simulink model "gm_test_cost_function_only_without_delays"  (R2022a)
settings: Solver=FixedStepDiscrete  StartTime=0.0  StopTime=10.0  RelTol=1e-3
undefined symbols (not defined in the file or in its folder): f_c
libraries: hdlmdlgenlib x64
(part 2 of 2)

== system gm_test_cost_function_only_without_delays/HDL_DUT1/Subsystem/Subsystem4 ==
  Prediction_5 : Inport  OutDataTypeStr=fixdt(1, 18, 11)  PortDimensions=[4]  SampleTime=1e-08
  id_ref : Inport  Port=2  OutDataTypeStr=fixdt(1, 18, 11)  PortDimensions=1  SampleTime=1e-08
  iq_ref : Inport  Port=3  OutDataTypeStr=fixdt(1, 18, 11)  PortDimensions=1  SampleTime=1e-08
  ix_ref : Inport  Port=4  OutDataTypeStr=fixdt(1, 18, 11)  PortDimensions=1  SampleTime=1e-08
  iy_ref : Inport  Port=5  OutDataTypeStr=fixdt(1, 18, 11)  PortDimensions=1  SampleTime=1e-08
  Prediction_5_0_wire : hdlmdlgenlib/Buffer
      settings: SourceProductBaseCode=SL
  Prediction_5_1_wire : hdlmdlgenlib/Buffer
      settings: SourceProductBaseCode=SL
  Prediction_5_2_wire : hdlmdlgenlib/Buffer
      settings: SourceProductBaseCode=SL
  Prediction_5_3_wire : hdlmdlgenlib/Buffer
      settings: SourceProductBaseCode=SL
  Product{1..4} (4 alike) : Product  Inputs=**  OutDataTypeStr=fixdt(1, 20, 11)  SampleTime=1e-08
  Subtract{4..7} (4 alike) : Sum  Inputs=+-  AccumDataTypeStr=fixdt(1, 19, 11)  OutDataTypeStr=fixdt(1, 20, 11)  SampleTime=1e-08
  Sum of Elements_stage2 : Sum  AccumDataTypeStr=fixdt(1, 22, 11)  OutDataTypeStr=fixdt(1, 21, 11)  SampleTime=1e-08
  Sum of Elements_stage3 : Sum  AccumDataTypeStr=fixdt(1, 22, 11)  OutDataTypeStr=fixdt(1, 22, 11)  SampleTime=1e-08
  Sum of Elements_stage4 : Sum  AccumDataTypeStr=fixdt(1, 22, 11)  OutDataTypeStr=fixdt(1, 20, 11)  SampleTime=1e-08
  t : Demux
  J5 : Outport  SampleTime=1e-08
  wires:
  Prediction_5/1 -> t/1
  id_ref/1 -> Subtract4/1
  iq_ref/1 -> Subtract5/1
  ix_ref/1 -> Subtract6/1
  iy_ref/1 -> Subtract7/1
  Prediction_5_0_wire/1 -> Subtract4/2
  Prediction_5_1_wire/1 -> Subtract5/2
  Prediction_5_2_wire/1 -> Subtract6/2
  Prediction_5_3_wire/1 -> Subtract7/2
  Product1/1 -> Sum of Elements_stage2/2
  Product2/1 -> Sum of Elements_stage3/2
  Product3/1 -> Sum of Elements_stage2/1
  Product4/1 -> Sum of Elements_stage4/2
  Subtract4/1 -> Product3/2, Product3/1
  Subtract5/1 -> Product1/2, Product1/1
  Subtract6/1 -> Product2/2, Product2/1
  Subtract7/1 -> Product4/2, Product4/1
  Sum of Elements_stage4/1 -> J5/1
  t/1 -> Prediction_5_0_wire/1
  t/2 -> Prediction_5_1_wire/1
  t/3 -> Prediction_5_2_wire/1
  t/4 -> Prediction_5_3_wire/1
  Sum of Elements_stage2/1 -> Sum of Elements_stage3/1
  Sum of Elements_stage3/1 -> Sum of Elements_stage4/1

== system gm_test_cost_function_only_without_delays/HDL_DUT1/Subsystem/Subsystem5 ==
  Prediction_6 : Inport  OutDataTypeStr=fixdt(1, 18, 11)  PortDimensions=[4]  SampleTime=1e-08
  id_ref : Inport  Port=2  OutDataTypeStr=fixdt(1, 18, 11)  PortDimensions=1  SampleTime=1e-08
  iq_ref : Inport  Port=3  OutDataTypeStr=fixdt(1, 18, 11)  PortDimensions=1  SampleTime=1e-08
  ix_ref : Inport  Port=4  OutDataTypeStr=fixdt(1, 18, 11)  PortDimensions=1  SampleTime=1e-08
  iy_ref : Inport  Port=5  OutDataTypeStr=fixdt(1, 18, 11)  PortDimensions=1  SampleTime=1e-08
  Prediction_6_0_wire : hdlmdlgenlib/Buffer
      settings: SourceProductBaseCode=SL
  Prediction_6_1_wire : hdlmdlgenlib/Buffer
      settings: SourceProductBaseCode=SL
  Prediction_6_2_wire : hdlmdlgenlib/Buffer
      settings: SourceProductBaseCode=SL
  Prediction_6_3_wire : hdlmdlgenlib/Buffer
      settings: SourceProductBaseCode=SL
  Product{1..4} (4 alike) : Product  Inputs=**  OutDataTypeStr=fixdt(1, 20, 11)  SampleTime=1e-08
  Subtract{4..7} (4 alike) : Sum  Inputs=+-  AccumDataTypeStr=fixdt(1, 19, 11)  OutDataTypeStr=fixdt(1, 20, 11)  SampleTime=1e-08
  Sum of Elements_stage2 : Sum  AccumDataTypeStr=fixdt(1, 22, 11)  OutDataTypeStr=fixdt(1, 21, 11)  SampleTime=1e-08
  Sum of Elements_stage3 : Sum  AccumDataTypeStr=fixdt(1, 22, 11)  OutDataTypeStr=fixdt(1, 22, 11)  SampleTime=1e-08
  Sum of Elements_stage4 : Sum  AccumDataTypeStr=fixdt(1, 22, 11)  OutDataTypeStr=fixdt(1, 20, 11)  SampleTime=1e-08
  t : Demux
  J6 : Outport  SampleTime=1e-08
  wires:
  Prediction_6/1 -> t/1
  id_ref/1 -> Subtract4/1
  iq_ref/1 -> Subtract5/1
  ix_ref/1 -> Subtract6/1
  iy_ref/1 -> Subtract7/1
  Prediction_6_0_wire/1 -> Subtract4/2
  Prediction_6_1_wire/1 -> Subtract5/2
  Prediction_6_2_wire/1 -> Subtract6/2
  Prediction_6_3_wire/1 -> Subtract7/2
  Product1/1 -> Sum of Elements_stage2/2
  Product2/1 -> Sum of Elements_stage3/2
  Product3/1 -> Sum of Elements_stage2/1
  Product4/1 -> Sum of Elements_stage4/2
  Subtract4/1 -> Product3/2, Product3/1
  Subtract5/1 -> Product1/2, Product1/1
  Subtract6/1 -> Product2/2, Product2/1
  Subtract7/1 -> Product4/2, Product4/1
  Sum of Elements_stage4/1 -> J6/1
  t/1 -> Prediction_6_0_wire/1
  t/2 -> Prediction_6_1_wire/1
  t/3 -> Prediction_6_2_wire/1
  t/4 -> Prediction_6_3_wire/1
  Sum of Elements_stage2/1 -> Sum of Elements_stage3/1
  Sum of Elements_stage3/1 -> Sum of Elements_stage4/1

== system gm_test_cost_function_only_without_delays/HDL_DUT1/Subsystem/Subsystem6 ==
  Prediction_7 : Inport  OutDataTypeStr=fixdt(1, 18, 11)  PortDimensions=[4]  SampleTime=1e-08
  id_ref : Inport  Port=2  OutDataTypeStr=fixdt(1, 18, 11)  PortDimensions=1  SampleTime=1e-08
  iq_ref : Inport  Port=3  OutDataTypeStr=fixdt(1, 18, 11)  PortDimensions=1  SampleTime=1e-08
  ix_ref : Inport  Port=4  OutDataTypeStr=fixdt(1, 18, 11)  PortDimensions=1  SampleTime=1e-08
  iy_ref : Inport  Port=5  OutDataTypeStr=fixdt(1, 18, 11)  PortDimensions=1  SampleTime=1e-08
  Prediction_7_0_wire : hdlmdlgenlib/Buffer
      settings: SourceProductBaseCode=SL
  Prediction_7_1_wire : hdlmdlgenlib/Buffer
      settings: SourceProductBaseCode=SL
  Prediction_7_2_wire : hdlmdlgenlib/Buffer
      settings: SourceProductBaseCode=SL
  Prediction_7_3_wire : hdlmdlgenlib/Buffer
      settings: SourceProductBaseCode=SL
  Product{1..4} (4 alike) : Product  Inputs=**  OutDataTypeStr=fixdt(1, 20, 11)  SampleTime=1e-08
  Subtract{4..7} (4 alike) : Sum  Inputs=+-  AccumDataTypeStr=fixdt(1, 19, 11)  OutDataTypeStr=fixdt(1, 20, 11)  SampleTime=1e-08
  Sum of Elements_stage2 : Sum  AccumDataTypeStr=fixdt(1, 22, 11)  OutDataTypeStr=fixdt(1, 21, 11)  SampleTime=1e-08
  Sum of Elements_stage3 : Sum  AccumDataTypeStr=fixdt(1, 22, 11)  OutDataTypeStr=fixdt(1, 22, 11)  SampleTime=1e-08
  Sum of Elements_stage4 : Sum  AccumDataTypeStr=fixdt(1, 22, 11)  OutDataTypeStr=fixdt(1, 20, 11)  SampleTime=1e-08
  t : Demux
  J7 : Outport  SampleTime=1e-08
  wires:
  Prediction_7/1 -> t/1
  id_ref/1 -> Subtract4/1
  iq_ref/1 -> Subtract5/1
  ix_ref/1 -> Subtract6/1
  iy_ref/1 -> Subtract7/1
  Prediction_7_0_wire/1 -> Subtract4/2
  Prediction_7_1_wire/1 -> Subtract5/2
  Prediction_7_2_wire/1 -> Subtract6/2
  Prediction_7_3_wire/1 -> Subtract7/2
  Product1/1 -> Sum of Elements_stage2/2
  Product2/1 -> Sum of Elements_stage3/2
  Product3/1 -> Sum of Elements_stage2/1
  Product4/1 -> Sum of Elements_stage4/2
  Subtract4/1 -> Product3/2, Product3/1
  Subtract5/1 -> Product1/2, Product1/1
  Subtract6/1 -> Product2/2, Product2/1
  Subtract7/1 -> Product4/2, Product4/1
  Sum of Elements_stage4/1 -> J7/1
  t/1 -> Prediction_7_0_wire/1
  t/2 -> Prediction_7_1_wire/1
  t/3 -> Prediction_7_2_wire/1
  t/4 -> Prediction_7_3_wire/1
  Sum of Elements_stage2/1 -> Sum of Elements_stage3/1
  Sum of Elements_stage3/1 -> Sum of Elements_stage4/1

== system gm_test_cost_function_only_without_delays/HDL_DUT1/Subsystem/Subsystem7 ==
  Prediction_8 : Inport  OutDataTypeStr=fixdt(1, 18, 11)  PortDimensions=[4]  SampleTime=1e-08
  id_ref : Inport  Port=2  OutDataTypeStr=fixdt(1, 18, 11)  PortDimensions=1  SampleTime=1e-08
  iq_ref : Inport  Port=3  OutDataTypeStr=fixdt(1, 18, 11)  PortDimensions=1  SampleTime=1e-08
  ix_ref : Inport  Port=4  OutDataTypeStr=fixdt(1, 18, 11)  PortDimensions=1  SampleTime=1e-08
  iy_ref : Inport  Port=5  OutDataTypeStr=fixdt(1, 18, 11)  PortDimensions=1  SampleTime=1e-08
  Prediction_8_0_wire : hdlmdlgenlib/Buffer
      settings: SourceProductBaseCode=SL
  Prediction_8_1_wire : hdlmdlgenlib/Buffer
      settings: SourceProductBaseCode=SL
  Prediction_8_2_wire : hdlmdlgenlib/Buffer
      settings: SourceProductBaseCode=SL
  Prediction_8_3_wire : hdlmdlgenlib/Buffer
      settings: SourceProductBaseCode=SL
  Product{1..4} (4 alike) : Product  Inputs=**  OutDataTypeStr=fixdt(1, 20, 11)  SampleTime=1e-08
  Subtract{4..7} (4 alike) : Sum  Inputs=+-  AccumDataTypeStr=fixdt(1, 19, 11)  OutDataTypeStr=fixdt(1, 20, 11)  SampleTime=1e-08
  Sum of Elements_stage2 : Sum  AccumDataTypeStr=fixdt(1, 22, 11)  OutDataTypeStr=fixdt(1, 21, 11)  SampleTime=1e-08
  Sum of Elements_stage3 : Sum  AccumDataTypeStr=fixdt(1, 22, 11)  OutDataTypeStr=fixdt(1, 22, 11)  SampleTime=1e-08
  Sum of Elements_stage4 : Sum  AccumDataTypeStr=fixdt(1, 22, 11)  OutDataTypeStr=fixdt(1, 20, 11)  SampleTime=1e-08
  t : Demux
  J8 : Outport  SampleTime=1e-08
  wires:
  Prediction_8/1 -> t/1
  id_ref/1 -> Subtract4/1
  iq_ref/1 -> Subtract5/1
  ix_ref/1 -> Subtract6/1
  iy_ref/1 -> Subtract7/1
  Prediction_8_0_wire/1 -> Subtract4/2
  Prediction_8_1_wire/1 -> Subtract5/2
  Prediction_8_2_wire/1 -> Subtract6/2
  Prediction_8_3_wire/1 -> Subtract7/2
  Product1/1 -> Sum of Elements_stage2/2
  Product2/1 -> Sum of Elements_stage3/2
  Product3/1 -> Sum of Elements_stage2/1
  Product4/1 -> Sum of Elements_stage4/2
  Subtract4/1 -> Product3/2, Product3/1
  Subtract5/1 -> Product1/2, Product1/1
  Subtract6/1 -> Product2/2, Product2/1
  Subtract7/1 -> Product4/2, Product4/1
  Sum of Elements_stage4/1 -> J8/1
  t/1 -> Prediction_8_0_wire/1
  t/2 -> Prediction_8_1_wire/1
  t/3 -> Prediction_8_2_wire/1
  t/4 -> Prediction_8_3_wire/1
  Sum of Elements_stage2/1 -> Sum of Elements_stage3/1
  Sum of Elements_stage3/1 -> Sum of Elements_stage4/1

== system gm_test_cost_function_only_without_delays/HDL_DUT1/Subsystem/Subsystem8 ==
  Prediction_9 : Inport  OutDataTypeStr=fixdt(1, 18, 11)  PortDimensions=[4]  SampleTime=1e-08
  id_ref : Inport  Port=2  OutDataTypeStr=fixdt(1, 18, 11)  PortDimensions=1  SampleTime=1e-08
  iq_ref : Inport  Port=3  OutDataTypeStr=fixdt(1, 18, 11)  PortDimensions=1  SampleTime=1e-08
  ix_ref : Inport  Port=4  OutDataTypeStr=fixdt(1, 18, 11)  PortDimensions=1  SampleTime=1e-08
  iy_ref : Inport  Port=5  OutDataTypeStr=fixdt(1, 18, 11)  PortDimensions=1  SampleTime=1e-08
  Prediction_9_0_wire : hdlmdlgenlib/Buffer
      settings: SourceProductBaseCode=SL
  Prediction_9_1_wire : hdlmdlgenlib/Buffer
      settings: SourceProductBaseCode=SL
  Prediction_9_2_wire : hdlmdlgenlib/Buffer
      settings: SourceProductBaseCode=SL
  Prediction_9_3_wire : hdlmdlgenlib/Buffer
      settings: SourceProductBaseCode=SL
  Product{1..4} (4 alike) : Product  Inputs=**  OutDataTypeStr=fixdt(1, 20, 11)  SampleTime=1e-08
  Subtract{4..7} (4 alike) : Sum  Inputs=+-  AccumDataTypeStr=fixdt(1, 19, 11)  OutDataTypeStr=fixdt(1, 20, 11)  SampleTime=1e-08
  Sum of Elements_stage2 : Sum  AccumDataTypeStr=fixdt(1, 22, 11)  OutDataTypeStr=fixdt(1, 21, 11)  SampleTime=1e-08
  Sum of Elements_stage3 : Sum  AccumDataTypeStr=fixdt(1, 22, 11)  OutDataTypeStr=fixdt(1, 22, 11)  SampleTime=1e-08
  Sum of Elements_stage4 : Sum  AccumDataTypeStr=fixdt(1, 22, 11)  OutDataTypeStr=fixdt(1, 20, 11)  SampleTime=1e-08
  t : Demux
  J9 : Outport  SampleTime=1e-08
  wires:
  Prediction_9/1 -> t/1
  id_ref/1 -> Subtract4/1
  iq_ref/1 -> Subtract5/1
  ix_ref/1 -> Subtract6/1
  iy_ref/1 -> Subtract7/1
  Prediction_9_0_wire/1 -> Subtract4/2
  Prediction_9_1_wire/1 -> Subtract5/2
  Prediction_9_2_wire/1 -> Subtract6/2
  Prediction_9_3_wire/1 -> Subtract7/2
  Product1/1 -> Sum of Elements_stage2/2
  Product2/1 -> Sum of Elements_stage3/2
  Product3/1 -> Sum of Elements_stage2/1
  Product4/1 -> Sum of Elements_stage4/2
  Subtract4/1 -> Product3/2, Product3/1
  Subtract5/1 -> Product1/2, Product1/1
  Subtract6/1 -> Product2/2, Product2/1
  Subtract7/1 -> Product4/2, Product4/1
  Sum of Elements_stage4/1 -> J9/1
  t/1 -> Prediction_9_0_wire/1
  t/2 -> Prediction_9_1_wire/1
  t/3 -> Prediction_9_2_wire/1
  t/4 -> Prediction_9_3_wire/1
  Sum of Elements_stage2/1 -> Sum of Elements_stage3/1
  Sum of Elements_stage3/1 -> Sum of Elements_stage4/1

== system gm_test_cost_function_only_without_delays/HDL_DUT1/Subsystem/Subsystem9 ==
  Prediction_10 : Inport  OutDataTypeStr=fixdt(1, 18, 11)  PortDimensions=[4]  SampleTime=1e-08
  id_ref : Inport  Port=2  OutDataTypeStr=fixdt(1, 18, 11)  PortDimensions=1  SampleTime=1e-08
  iq_ref : Inport  Port=3  OutDataTypeStr=fixdt(1, 18, 11)  PortDimensions=1  SampleTime=1e-08
  ix_ref : Inport  Port=4  OutDataTypeStr=fixdt(1, 18, 11)  PortDimensions=1  SampleTime=1e-08
  iy_ref : Inport  Port=5  OutDataTypeStr=fixdt(1, 18, 11)  PortDimensions=1  SampleTime=1e-08
  Prediction_10_0_wire : hdlmdlgenlib/Buffer
      settings: SourceProductBaseCode=SL
  Prediction_10_1_wire : hdlmdlgenlib/Buffer
      settings: SourceProductBaseCode=SL
  Prediction_10_2_wire : hdlmdlgenlib/Buffer
      settings: SourceProductBaseCode=SL
  Prediction_10_3_wire : hdlmdlgenlib/Buffer
      settings: SourceProductBaseCode=SL
  Product{1..4} (4 alike) : Product  Inputs=**  OutDataTypeStr=fixdt(1, 20, 11)  SampleTime=1e-08
  Subtract{4..7} (4 alike) : Sum  Inputs=+-  AccumDataTypeStr=fixdt(1, 19, 11)  OutDataTypeStr=fixdt(1, 20, 11)  SampleTime=1e-08
  Sum of Elements_stage2 : Sum  AccumDataTypeStr=fixdt(1, 22, 11)  OutDataTypeStr=fixdt(1, 21, 11)  SampleTime=1e-08
  Sum of Elements_stage3 : Sum  AccumDataTypeStr=fixdt(1, 22, 11)  OutDataTypeStr=fixdt(1, 22, 11)  SampleTime=1e-08
  Sum of Elements_stage4 : Sum  AccumDataTypeStr=fixdt(1, 22, 11)  OutDataTypeStr=fixdt(1, 20, 11)  SampleTime=1e-08
  t : Demux
  J10 : Outport  SampleTime=1e-08
  wires:
  Prediction_10/1 -> t/1
  id_ref/1 -> Subtract4/1
  iq_ref/1 -> Subtract5/1
  ix_ref/1 -> Subtract6/1
  iy_ref/1 -> Subtract7/1
  Prediction_10_0_wire/1 -> Subtract4/2
  Prediction_10_1_wire/1 -> Subtract5/2
  Prediction_10_2_wire/1 -> Subtract6/2
  Prediction_10_3_wire/1 -> Subtract7/2
  Product1/1 -> Sum of Elements_stage2/2
  Product2/1 -> Sum of Elements_stage3/2
  Product3/1 -> Sum of Elements_stage2/1
  Product4/1 -> Sum of Elements_stage4/2
  Subtract4/1 -> Product3/2, Product3/1
  Subtract5/1 -> Product1/2, Product1/1
  Subtract6/1 -> Product2/2, Product2/1
  Subtract7/1 -> Product4/2, Product4/1
  Sum of Elements_stage4/1 -> J10/1
  t/1 -> Prediction_10_0_wire/1
  t/2 -> Prediction_10_1_wire/1
  t/3 -> Prediction_10_2_wire/1
  t/4 -> Prediction_10_3_wire/1
  Sum of Elements_stage2/1 -> Sum of Elements_stage3/1
  Sum of Elements_stage3/1 -> Sum of Elements_stage4/1
